simulink model "Project"  (R2023b)
settings: Solver=FixedStepAuto  StartTime=0.0  StopTime=0.02  FixedStep=0.000125  RelTol=1e-3
libraries: simulink x2
settings Model: Creator=sony  LastModifiedBy=User

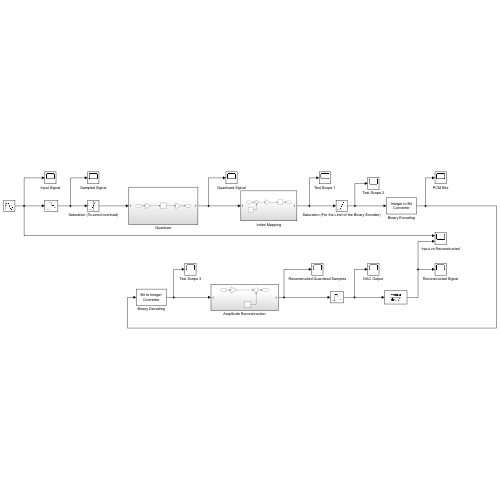
[thumbnail: Simulink's stored preview of the top-level diagram]
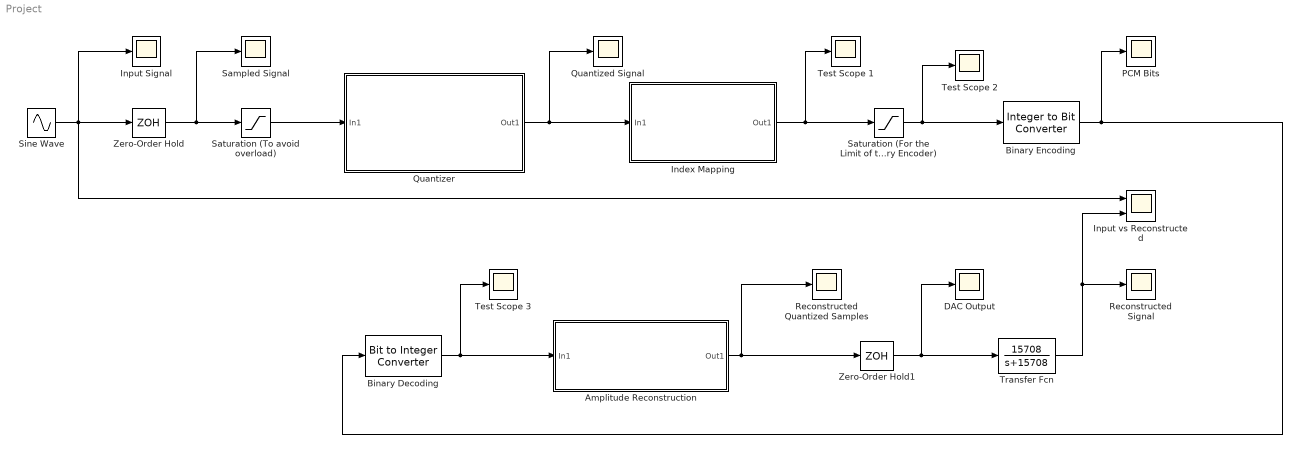
== system Project ==
  Amplitude Reconstruction : Subsystem
  Binary Decoding : simulink/Logic and Bit Operations/Bit to Integer Converter  nbits=8  bitOrder=MSB first  signedOutputValues=Unsigned  outDtype=Inherit via internal rule  outDtypeSigned=Inherit via internal rule
  Binary Encoding : simulink/Logic and Bit Operations/Integer to Bit Converter  nbits=8  signedInputValues=Unsigned  bitOrder=MSB first  outDtype=Inherit via internal rule
  DAC Output : Scope
  Index Mapping : Subsystem
  Input Signal : Scope
  Input vs Reconstructed : Scope  NumInputPorts=2
  PCM Bits : Scope
  Quantized Signal : Scope
  Quantizer : Subsystem
  Reconstructed Quantized Samples : Scope
  Reconstructed Signal : Scope
  Sampled Signal : Scope
  Saturation (For the Limit of the Binary Encoder) : Saturate  UpperLimit=255  LowerLimit=0
  Saturation (To avoid overload) : Saturate  UpperLimit=+2  LowerLimit=-2
  Sine Wave : Sin  Amplitude=2  Frequency=2*pi*950  SampleTime=0
  Test Scope 1 : Scope
  Test Scope 2 : Scope
  Test Scope 3 : Scope
  Transfer Fcn : TransferFcn  Numerator=[15708]  Denominator=[1 15708]
  Zero-Order Hold : ZeroOrderHold  SampleTime=0.000125
  Zero-Order Hold1 : ZeroOrderHold  SampleTime=0.000125
  wires:
  Sine Wave/1 -> Input vs Reconstructed/1, Zero-Order Hold/1, Input Signal/1
  Zero-Order Hold/1 -> Saturation (To avoid overload)/1, Sampled Signal/1
  Saturation (To avoid overload)/1 -> Quantizer/1(In1)
  Quantizer/1(Out1) -> Index Mapping/1(In1), Quantized Signal/1
  Binary Encoding/1 -> Binary Decoding/1, PCM Bits/1
  Saturation (For the Limit of the Binary Encoder)/1 -> Binary Encoding/1, Test Scope 2/1
  Index Mapping/1(Out1) -> Test Scope 1/1, Saturation (For the Limit of the Binary Encoder)/1
  Binary Decoding/1 -> Amplitude Reconstruction/1(In1), Test Scope 3/1
  Amplitude Reconstruction/1(Out1) -> Zero-Order Hold1/1, Reconstructed Quantized Samples/1
  Zero-Order Hold1/1 -> Transfer Fcn/1, DAC Output/1
  Transfer Fcn/1 -> Input vs Reconstructed/2, Reconstructed Signal/1

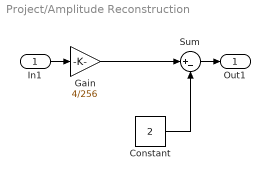
== system Project/Amplitude Reconstruction ==
  In1 : Inport
  Constant : Constant  Value=2
  Gain : Gain  Gain=4/256
  Sum : Sum  Inputs=|+-
  Out1 : Outport
  wires:
  Constant/1 -> Sum/2
  Gain/1 -> Sum/1
  Sum/1 -> Out1/1
  In1/1 -> Gain/1

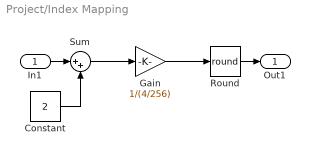
== system Project/Index Mapping ==
  In1 : Inport
  Constant : Constant  Value=2
  Gain : Gain  Gain=1/(4/256)
  Round : Rounding  Operator=round
  Sum : Sum  Inputs=|++
  Out1 : Outport
  wires:
  Sum/1 -> Gain/1
  Constant/1 -> Sum/2
  In1/1 -> Sum/1
  Gain/1 -> Round/1
  Round/1 -> Out1/1

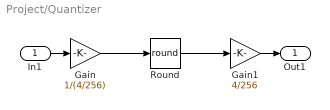
== system Project/Quantizer ==
  In1 : Inport
  Gain : Gain  Gain=1/(4/256)
  Gain1 : Gain  Gain=4/256
  Round : Rounding  Operator=round
  Out1 : Outport
  wires:
  Round/1 -> Gain1/1
  Gain/1 -> Round/1
  Gain1/1 -> Out1/1
  In1/1 -> Gain/1
